simulink model "G20_final_5bus_System"  (R2021a)
settings: Solver=VariableStepAuto  StartTime=0.0  StopTime=1  MaxStep=1e-4  RelTol=1e-3  EnableMultiTasking=on
libraries: neural x105, spsThreePhaseSeriesRLCBranchLib x27, spsGroundLib x10, spsThreePhaseVIMeasurementLib x5, spsLoadFlowBusLib x5, spsThreePhaseSeriesRLCLoadLib x4, spsThreePhaseSourceLib x2, spsCurrentMeasurementLib x1, spsThreePhaseFaultLib x1, spspowerguiLib x1
(part 3 of 3)

== system G20_final_5bus_System/Function Fitting Neural Network/Layer 2/Delays 1 ==
  "p{2}" : Inport  PortDimensions=100
      mask Display: e = 0.06;c1 = [120 230 180]/255;c2 = ([120 230 180]+0)/(256+128);c3 = ([120 230 180]+128)/(256+128);patch([0 1 1 0],[0 0 1 1],c1);patch([0 1 1 1-e 1-e 0+e],[0 0 1 1-e 0+e 0+e],c2);patch([0 0 1 1-e 0+e 0+e],[0 1 1 1-e 1-e 0+e],c3);plot([0 1 1 0 0],[0 0 1 1 0]);
  mux : Mux  Inputs=1
      mask Display: e = 0.06;c1 = [120 150 230]/255;c2 = ([120 150 230]+0)/383;c3 = ([120 150 230]+128)/383;patch([0 1 1 0],[0 0 1 1],c1);patch([0 1 1 1-e 1-e 0+e],[0 0 1 1-e 0+e 0+e],c2);patch([0 0 1 1-e 0+e 0+e],[0 1 1 1-e 1-e 0+e],c3);plot([0 1 1 0 0],[0 0 1 1 0]);disp('Mux')
  "pd{2,1}" : Outport
      mask Display: e = 0.06;c1 = [120 230 180]/255;c2 = ([120 230 180]+0)/(256+128);c3 = ([120 230 180]+128)/(256+128);patch([0 1 1 0],[0 0 1 1],c1);patch([0 1 1 1-e 1-e 0+e],[0 0 1 1-e 0+e 0+e],c2);patch([0 0 1 1-e 0+e 0+e],[0 1 1 1-e 1-e 0+e],c3);plot([0 1 1 0 0],[0 0 1 1 0]);
  wires:
  "p{2}"/1 -> mux/1
  mux/1 -> "pd{2,1}"/1

== system G20_final_5bus_System/Function Fitting Neural Network/Layer 2/LW{2,1} ==
  "ad{2,1}" : Inport  PortDimensions=100
      mask Display: e = 0.06;c1 = [120 230 180]/255;c2 = ([120 230 180]+0)/(256+128);c3 = ([120 230 180]+128)/(256+128);patch([0 1 1 0],[0 0 1 1],c1);patch([0 1 1 1-e 1-e 0+e],[0 0 1 1-e 0+e 0+e],c2);patch([0 0 1 1-e 0+e 0+e],[0 1 1 1-e 1-e 0+e],c3);plot([0 1 1 0 0],[0 0 1 1 0]);
  "IW{2,1}(1,:)'" : Constant  Value=[-0.1922792687813241752081694357912056148052215576171875;-0.1643782503465060773617523182110744528472423553466796875;-0.2140464150662836628757901280550868250429630279541015625;0.64984237530685129424767865202738903462886810302734375;0.06515173160389332862596489803763688541948795318603515625;0.32428565109393048260244540870189666748046875;0.44664615163111920370653251666226424276828765869140625;-0.5416359429188639662555715403868816792964935302734375;0.08451010338189375581396944880907540209591388702392578125;-0.68085104173427357654446723245200701057910919189453125;0.74411649049647710096877517571556381881237030029296875;-0.63444910715048663529813666173140518367290496826171875;0.26191560616716091924871534502017311751842498779296875;0.416031539955069751268723621251410804688930511474609375;0.7399917354728200447055996846756897866725921630859375;-0.50570164130127237545053731082589365541934967041015625;-0.6330968448110454449562212175806052982807159423828125;0.3931172695238800418593427821178920567035675048828125;-0.7474420670647539122199987104977481067180633544921875;0.692329261360826730964390662848018109798431396484375;-0.1833300597736831349937602908539702184498310089111328125;-0.41563548735982080994943999030510894954204559326171875;-0.67783894125960275633957508034654892981052398681640625;0.9240081508494852879920244959066621959209442138671875;0.306697590622211080368941793494741432368755340576171875;0.283746656566451205261358836651197634637355804443359375;-0.6393412437560372918454731916426680982112884521484375;0.49427762253848772644460041192360222339630126953125;0.70547441193553483973488482661196030676364898681640625;0.253123833635440054212750737860915251076221466064453125;-0.76758760037915230167726576837594620883464813232421875;-0.92565556519488334519252248355769552290439605712890625;0.60231073192691841899915061731007881462574005126953125;-0.706474212477285590239262091927230358123779296875;-0.438840783383022292607478220816119574010372161865234375;0.3882997036925208700353095991886220872402191162109375;0.146487635174426367168365459292544983327388763427734375;-0.78269288411060455867840346400043927133083343505859375;0.302086659286136816060519549864693544805049896240234375;-0.0222645853694913194165128089707650360651314258575439453125;-0.03100634299316044895089561350687290541827678680419921875;0.0275502807183102584043243865608019405044615268707275390625;0.24621497469874042973714267645846121013164520263671875;0.2386558727027703052936402627892675809562206268310546875;-0.264328180141567781191724861855618655681610107421875;-0.0887262507152713764124740691840997897088527679443359375;-0.6019727511350279058888190775178372859954833984375;0.307459545520185895117748486882192082703113555908203125;-0.48295906272489208532761040260083973407745361328125;-0.318331312864034876586316613611415959894657135009765625;-0.345378458617436712163595302627072669565677642822265625;-0.1921445207563619306245783491249312646687030792236328125;-0.77569309397441543740825409258832223713397979736328125;0.1973634531380060452843139273682027123868465423583984375;0.235901742665117819530706810837727971374988555908203125;0.01539418833776769190979649692962993867695331573486328125;0.61230148959426633492597602526075206696987152099609375;-0.215808304860677591108242268091998994350433349609375;-0.6828187020066156520670119789429008960723876953125;-0.1966308042302177538918073196327895857393741607666015625;-0.472255586161041074344524304251535795629024505615234375;0.53272422376683359335203249429468996822834014892578125;-0.4803128406984493725673246444785036146640777587890625;0.19616125686699692476366863047587685286998748779296875;0.11327082841527424950101021750015206634998321533203125;-0.40067957409805343704789493131102062761783599853515625;0.12466333562862912109903135160493548028171062469482421875;-0.1475818446608633538463806189611204899847507476806640625;0.60481769977131205617837395038804970681667327880859375;0.05190005496872847345901647031496395356953144073486328125 ...(+1715 chars)]
      mask Display: e = 0.06;c1 = [120 150 230]/255;c2 = ([120 150 230]+0)/383;c3 = ([120 150 230]+128)/383;patch([0 1 1 0],[0 0 1 1],c1);patch([0 1 1 1-e 1-e 0+e],[0 0 1 1-e 0+e 0+e],c2);patch([0 0 1 1-e 0+e 0+e],[0 1 1 1-e 1-e 0+e],c3);plot([0 1 1 0 0],[0 0 1 1 0]);disp('weights');
  Mux : Mux  Inputs=1
      mask Display: e = 0.06;c1 = [120 150 230]/255;c2 = ([120 150 230]+0)/383;c3 = ([120 150 230]+128)/383;patch([0 1 1 0],[0 0 1 1],c1);patch([0 1 1 1-e 1-e 0+e],[0 0 1 1-e 0+e 0+e],c2);patch([0 0 1 1-e 0+e 0+e],[0 1 1 1-e 1-e 0+e],c3);plot([0 1 1 0 0],[0 0 1 1 0]);disp('Mux');
  dotprod1 : neural/Weight Functions/dotprod
  "lz{2,1}" : Outport
      mask Display: e = 0.06;c1 = [120 230 180]/255;c2 = ([120 230 180]+0)/(256+128);c3 = ([120 230 180]+128)/(256+128);patch([0 1 1 0],[0 0 1 1],c1);patch([0 1 1 1-e 1-e 0+e],[0 0 1 1-e 0+e 0+e],c2);patch([0 0 1 1-e 0+e 0+e],[0 1 1 1-e 1-e 0+e],c3);plot([0 1 1 0 0],[0 0 1 1 0]);
  wires:
  "IW{2,1}(1,:)'"/1 -> dotprod1/1
  "ad{2,1}"/1 -> dotprod1/2
  dotprod1/1 -> Mux/1
  Mux/1 -> "lz{2,1}"/1
